simulink library "ChimeSystemLibBtc"  (R2022b)
settings: Solver=VariableStepAuto  StartTime=0.0  StopTime=10.0  RelTol=1e-3
undefined symbols (not defined in the file or in its folder): chimeConfig
libraries: AnnVncBtc x1, NonEntGainCalcBtc x1, RTC x1, ExternalChimeProcessBtc x1, HandyTextFile x1, ScalarChimeControlLibBtc x1, WavePlayLibBtc x1
settings Model: Creator=kl13806  LastModifiedBy=kl13806
settings SolverCC: AlgebraicLoopSolver=TrustRegion
settings DebuggingCC: UnconnectedInputMsg=warning  UnconnectedOutputMsg=warning  UnconnectedLineMsg=warning  SFMachineParentedDataDiag=warning
settings ModelReferenceCC: EnableRefExpFcnMdlSchedulingChecks=on
settings RTWCC: DLArmComputeVersion=19.05

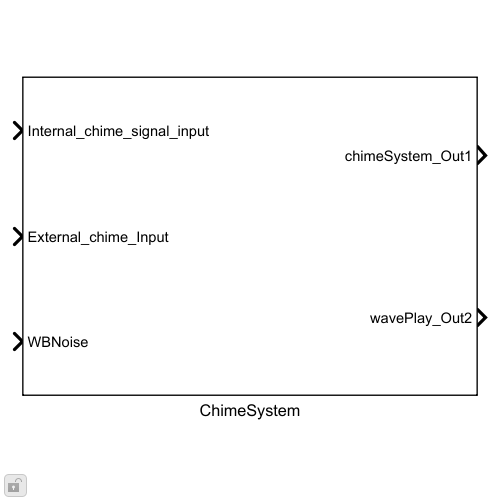
[thumbnail: Simulink's stored preview of the top-level diagram]
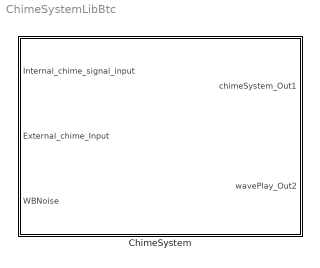
== system ChimeSystemLibBtc ==
  ChimeSystem : Subsystem  mask{Config=[]}
      mask prompts: Config "ChimeSystemConfig"
      mask init:
      | blkh=gcbh;
      | Config=BTConfig.Assert(blkh,Config);
      | 
      | Config.Validate();

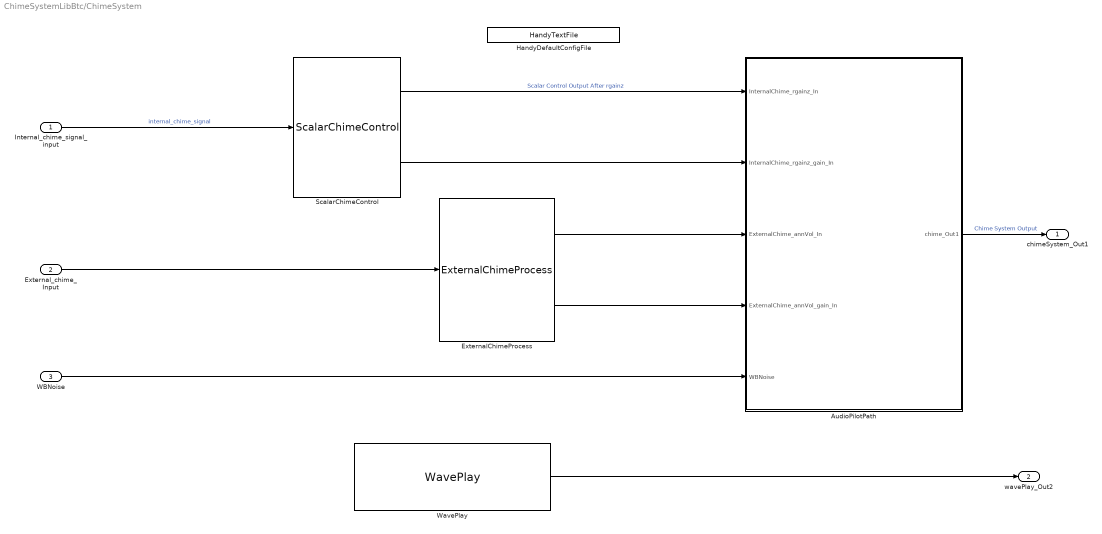
== system ChimeSystemLibBtc/ChimeSystem ==
  Internal_chime_signal_input : Inport
  External_chime_Input : Inport  Port=2
  WBNoise : Inport  Port=3
  AudioPilotPath : Subsystem
  ExternalChimeProcess : ExternalChimeProcessBtc/ExternalChimeProcess  Config=Config.ExternalChimeProcess
      settings: SourceProductName=Bose Blocklib
  HandyDefaultConfigFile : HandyTextFile/HandyTextFile  TemplateSource=Config  FileSuffix=Init  OpenDialogOnLoad=off  UseThisBlockName=off  TheDefaultText=|  ShowInLibBrowser=on
      | % $(FILENAME) Setup model parameters for each "Init" callback (e.g. update diagram)
      | sample_rate_in_hertz = 44100;
      | frame_size = 32;
      | sysin_channel_count = 2;
  ScalarChimeControl : ScalarChimeControlLibBtc/ScalarChimeControl  Config=Config
      settings: SourceProductName=Bose Blocklib
  WavePlay : WavePlayLibBtc/WavePlay  Config=Config.WavePlay  FeatureName=WavePlay
      settings: SourceProductName=Bose Blocklib
  chimeSystem_Out1 : Outport  VectorParamsAs1DForOutWhenUnconnected=off
  wavePlay_Out2 : Outport  Port=2  VectorParamsAs1DForOutWhenUnconnected=off
  wires:
  ScalarChimeControl/1 -> AudioPilotPath/1(InternalChime_rgainz_In)  "Scalar Control Output After rgainz"
  AudioPilotPath/1(chime_Out1) -> chimeSystem_Out1/1  "Chime System Output"
  Internal_chime_signal_input/1 -> ScalarChimeControl/1  "internal_chime_signal"
  ScalarChimeControl/2 -> AudioPilotPath/2(InternalChime_rgainz_gain_In)
  ExternalChimeProcess/1 -> AudioPilotPath/3(ExternalChime_annVol_In)
  ExternalChimeProcess/2 -> AudioPilotPath/4(ExternalChime_annVol_gain_In)
  WavePlay/1 -> wavePlay_Out2/1
  External_chime_Input/1 -> ExternalChimeProcess/1
  WBNoise/1 -> AudioPilotPath/5(WBNoise)

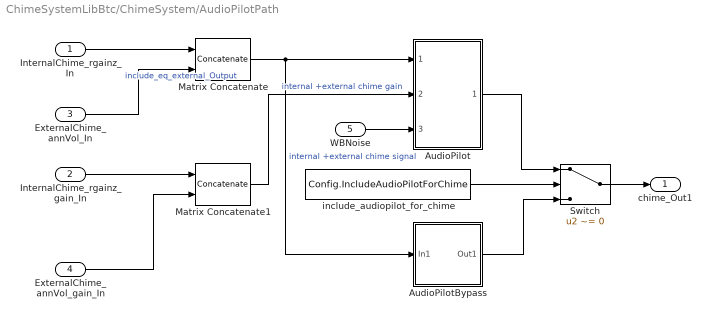
== system ChimeSystemLibBtc/ChimeSystem/AudioPilotPath ==
  InternalChime_rgainz_In : Inport
  InternalChime_rgainz_gain_In : Inport  Port=2
  ExternalChime_annVol_In : Inport  Port=3
  ExternalChime_annVol_gain_In : Inport  Port=4
  WBNoise : Inport  Port=5
  AudioPilot : Subsystem
  AudioPilotBypass : Subsystem
  Matrix Concatenate : Concatenate  Mode=Multidimensional array  ConcatenateDimension=2
  Matrix Concatenate1 : Concatenate  Mode=Multidimensional array  ConcatenateDimension=2
  Switch : Switch  Criteria=u2 ~= 0  SaturateOnIntegerOverflow=off  InputSameDT=off
  include_audiopilot_for_chime : Constant  Value=Config.IncludeAudioPilotForChime  VectorParams1D=off  OutDataTypeStr=single
  chime_Out1 : Outport  VectorParamsAs1DForOutWhenUnconnected=off
  wires:
  include_audiopilot_for_chime/1 -> Switch/2
  AudioPilotBypass/1(Out1) -> Switch/3
  AudioPilot/1(VncOut) -> Switch/1
  Matrix Concatenate1/1 -> AudioPilot/2(VolGain)  "internal +external chime gain"
  Matrix Concatenate/1 -> AudioPilotBypass/1(In1), AudioPilot/1(AudioIn)  "internal +external chime signal"
  ExternalChime_annVol_gain_In/1 -> Matrix Concatenate1/2
  InternalChime_rgainz_In/1 -> Matrix Concatenate/1
  ExternalChime_annVol_In/1 -> Matrix Concatenate/2  "include_eq_external_Output"
  InternalChime_rgainz_gain_In/1 -> Matrix Concatenate1/1
  Switch/1 -> chime_Out1/1
  WBNoise/1 -> AudioPilot/3(WBNoise)

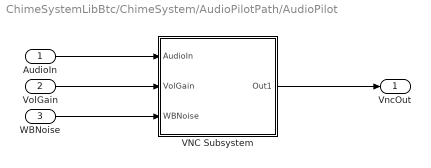
== system ChimeSystemLibBtc/ChimeSystem/AudioPilotPath/AudioPilot ==
  AudioIn : Inport
  VolGain : Inport  Port=2
  WBNoise : Inport  Port=3
  VNC Subsystem : Subsystem  TreatAsAtomicUnit=on
  VncOut : Outport  VectorParamsAs1DForOutWhenUnconnected=off
  wires:
  VNC Subsystem/1(Out1) -> VncOut/1
  VolGain/1 -> VNC Subsystem/2(VolGain)
  AudioIn/1 -> VNC Subsystem/1(AudioIn)
  WBNoise/1 -> VNC Subsystem/3(WBNoise)

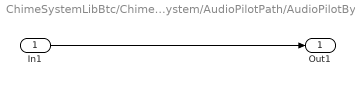
== system ChimeSystemLibBtc/ChimeSystem/AudioPilotPath/AudioPilotBypass ==
  In1 : Inport
  Out1 : Outport  VectorParamsAs1DForOutWhenUnconnected=off
  wires:
  In1/1 -> Out1/1

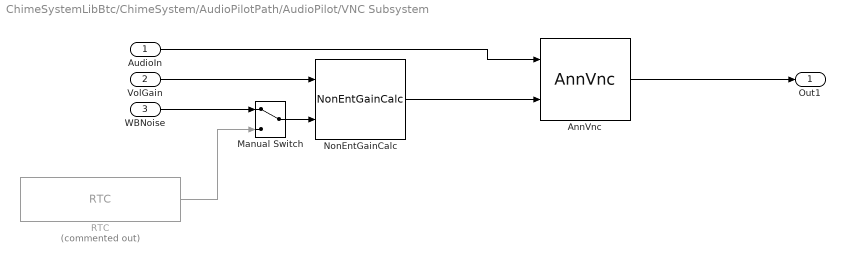
== system ChimeSystemLibBtc/ChimeSystem/AudioPilotPath/AudioPilot/VNC Subsystem ==
  AudioIn : Inport
  VolGain : Inport  Port=2
  WBNoise : Inport  Port=3
  AnnVnc : AnnVncBtc/AnnVnc  Config=Config.AnnVnc  FeatureName=AnnVnc
      settings: SourceProductName=Bose Blocklib
  Manual Switch : ManualSwitch
  NonEntGainCalc : NonEntGainCalcBtc/NonEntGainCalc  Config=Config.NonEntGainCalc  FeatureName=NonEntGainCalc
      settings: SourceProductName=Bose Blocklib
  RTC : RTC/RTC  Commented=on  REQ_Priority=RTC_Mask.NormalPriority  RequestAtInit=off  EnableRequest=off  REQElemName1=NoiseSig  REQElemType1=single  REQElemWidth1=length(chimeConfig.GainCalc.noise)  REQElemInitial1=[]  REQElemType2=uint32  REQElemWidth2=1  REQElemInitial2=[]  REQElemType3=uint32  REQElemWidth3=1  REQElemInitial3=[]  REQElemType4=uint32  REQElemWidth4=1  REQElemInitial4=[]  REQElemType5=uint32  REQElemWidth5=1  REQElemInitial5=[]  REQElemType6=uint32  REQElemWidth6=1  REQElemInitial6=[]  REQElemType7=uint32  REQElemWidth7=1  REQElemInitial7=[]  REQElemType8=uint32  REQElemWidth8=1  REQElemInitial8=[]  REQElemType9=uint32  REQElemWidth9=1  REQElemInitial9=[]  REQElemType10=uint32  REQElemWidth10=1  REQElemInitial10=[]  EnableResponse=on  EnableRSP_StatusIn=off  RSPElemType1=uint32  RSPElemWidth1=1  RSPElemType2=uint32  RSPElemWidth2=1  RSPElemType3=uint32  RSPElemWidth3=1  RSPElemType4=uint32  RSPElemWidth4=1  RSPElemType5=uint32  RSPElemWidth5=1  RSPElemType6=uint32  RSPElemWidth6=1  RSPElemType7=uint32  RSPElemWidth7=1  RSPElemType8=uint32  RSPElemWidth8=1  RSPElemType9=uint32  RSPElemWidth9=1  RSPElemType10=uint32  RSPElemWidth10=1  EnableNotification=off  EnableNTF_PrepTrig=off  NTFElemType1=uint32  NTFElemWidth1=1  NTFElemType2=uint32  NTFElemWidth2=1  NTFElemType3=uint32  NTFElemWidth3=1  NTFElemType4=uint32  NTFElemWidth4=1  NTFElemType5=uint32  NTFElemWidth5=1  NTFElemType6=uint32  NTFElemWidth6=1  NTFElemType7=uint32  NTFElemWidth7=1  NTFElemType8=uint32  NTFElemWidth8=1  NTFElemType9=uint32  NTFElemWidth9=1  NTFElemType10=uint32  NTFElemWidth10=1  MaskMessageName=VNCNoiseSig
  Out1 : Outport  VectorParamsAs1DForOutWhenUnconnected=off
  wires:
  VolGain/1 -> NonEntGainCalc/1
  AnnVnc/1 -> Out1/1
  AudioIn/1 -> AnnVnc/1
  NonEntGainCalc/1 -> AnnVnc/2
  WBNoise/1 -> Manual Switch/1
  Manual Switch/1 -> NonEntGainCalc/2
  RTC/1 -> Manual Switch/2
